simulink model "Simulink_transfer"  (R2017a)
settings: Solver=VariableStepAuto  StartTime=0.0  StopTime=10.0  RelTol=1e-3
undefined symbols (not defined in the file or in its folder): G
settings Model: Creator=medlem  LastModifiedBy=Oystein

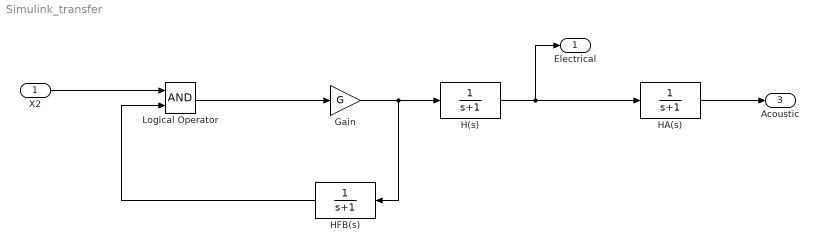
== system Simulink_transfer ==
  X2 : Inport
  Gain : Gain  Gain=G
  H(s) : TransferFcn  Denominator=[1 1]
  HA(s) : TransferFcn  Denominator=[1 1]
  HFB(s) : TransferFcn  Denominator=[1 1]
  Logical Operator : Logic  AllPortsSameDT=off  OutDataTypeStr=boolean
  Electrical : Outport  SignalName=X7
  Acoustic : Outport  Port=3
  wires:
  Logical Operator/1 -> Gain/1
  X2/1 -> Logical Operator/1
  Gain/1 -> HFB(s)/1, H(s)/1
  HFB(s)/1 -> Logical Operator/2
  HA(s)/1 -> Acoustic/1
  H(s)/1 -> Electrical/1, HA(s)/1
